simulink model "MdXXArray"  (R2024b)
settings: Solver=FixedStepDiscrete  StartTime=0.0  StopTime=10.0  FixedStep=0.01  RelTol=1e-3
(part 2 of 2)

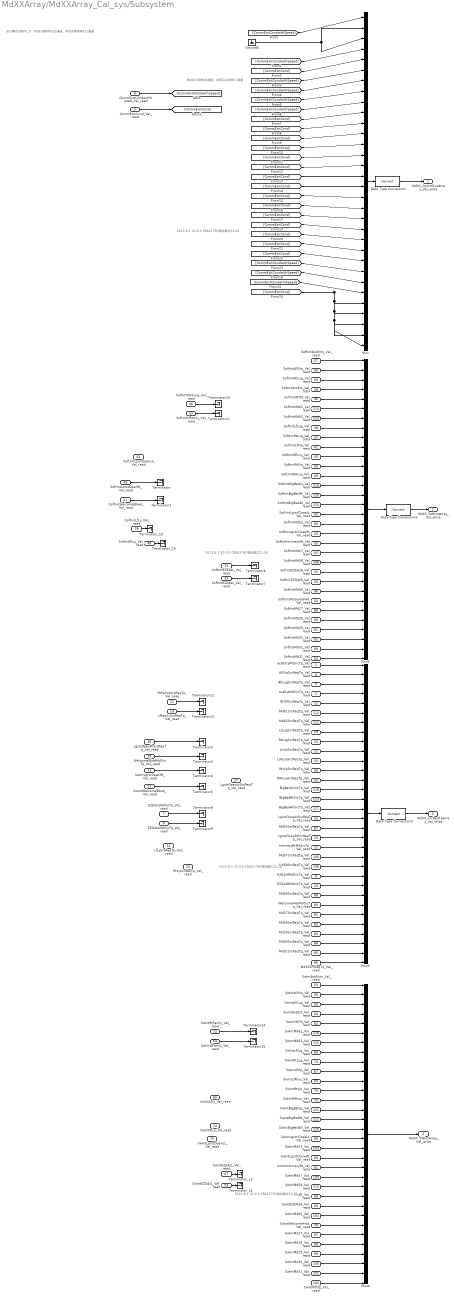
== system MdXXArray/MdXXArray_Cal_sys/Subsystem ==
  note: Md60占用Md6通道，Md61占用Md7通道
  note: 557模式流程V1.9：Md53借用Md18通道，Md56借用Md25通道
  note: 2023.8.1 V2.0.0 CR401790 增加模式21-26
  note: 2023.8.1 V2.0.0 CR401790 增加模式21-26
  note: 2023.8.1 V2.0.0 CR401790 增加模式21-26
  note: 2023.8.1 V2.0.0 CR421790 增加模式21-26
  acsEntyMdSrcTp_Val_read : Inport
  acsExtMdSrcTp_Val_read : Inport  Port=2
  AllLugSrcReqTp_Val_read : Inport  Port=3
  AllVipSrcReqTp_Val_read : Inport  Port=4
  CommExitCond_Val_read : Inport  Port=5
  CommExitCondwithSpeed_Val_read : Inport  Port=6
  EZE4sLMdSrcTp_Val_read : Inport  Port=7
  EZE4sRMdSrcTp_Val_read : Inport  Port=8
  EZQ4sLMdSrcTp_Val_read : Inport  Port=9
  EZQ4sRMdSrcTp_Val_read : Inport  Port=10
  IntimacyRtMdSrcTp_Val_read : Inport  Port=11
  INTMSrcReqTp_Val_read : Inport  Port=12
  LfFamlySrcReqTp_Val_read : Inport  Port=13
  LfLySrcReqTp_Val_read : Inport  Port=14
  LgrstCloseLtSrcReqTp_Val_read : Inport  Port=15
  LgrstCloseRtSrcReqTp_Val_read : Inport  Port=16
  LgrstOpenLtSrcReqTp_Val_read : Inport  Port=17
  LgrstOpenRtSrcReqTp_Val_read : Inport  Port=18
  LtLugSrcReqTp_Val_read : Inport  Port=19
  LtRcvySrcReqTp_Val_read : Inport  Port=20
  LtVipSrcReqTp_Val_read : Inport  Port=21
  RtFamlySrcReqTp_Val_read : Inport  Port=22
  RtLugSrcReqTp_Val_read : Inport  Port=23
  RtLySrcReqTp_Val_read : Inport  Port=24
  RtRcvySrcReqTp_Val_read : Inport  Port=25
  RtVipSrcReqTp_Val_read : Inport  Port=26
  SoftIntAcsEnty_Val_read : Inport  Port=27
  SoftIntAcsExt_Val_read : Inport  Port=28
  SoftIntAllLug_Val_read : Inport  Port=29
  SoftIntAllVip_Val_read : Inport  Port=30
  SoftIntEZE4sL_Val_read : Inport  Port=31
  SoftIntEZE4sR_Val_read : Inport  Port=32
  SoftIntEZQ4sL_Val_read : Inport  Port=33
  SoftIntEZQ4sR_Val_read : Inport  Port=34
  SoftIntIntimacyRt_Val_read : Inport  Port=35
  SoftIntINTM_Val_read : Inport  Port=36
  SoftIntLfFamly_Val_read : Inport  Port=37
  SoftIntLfLug_Val_read : Inport  Port=38
  SoftIntLfLy_Val_read : Inport  Port=39
  SoftIntLfRcvy_Val_read : Inport  Port=40
  SoftIntLfVip_Val_read : Inport  Port=41
  SoftIntLgrstCloseLt_Val_read : Inport  Port=42
  SoftIntLgrstCloseRt_Val_read : Inport  Port=43
  SoftIntLgrstOpenLt_Val_read : Inport  Port=44
  SoftIntLgrstOpenRt_Val_read : Inport  Port=45
  SoftIntRtFamly_Val_read : Inport  Port=46
  SoftIntRtLug_Val_read : Inport  Port=47
  SoftIntRtLy_Val_read : Inport  Port=48
  SoftIntRtRcvy_Val_read : Inport  Port=49
  SoftIntRtVip_Val_read : Inport  Port=50
  SoftIntWelcomeBkwd_Val_read : Inport  Port=51
  SoftIntWelcomeFwd_Val_read : Inport  Port=52
  SwIntAcsEnty_Val_read : Inport  Port=53
  SwIntAcsExt_Val_read : Inport  Port=54
  SwIntAllLug_Val_read : Inport  Port=55
  SwIntAllVip_Val_read : Inport  Port=56
  SwIntEZE4sL_Val_read : Inport  Port=57
  SwIntEZE4sR_Val_read : Inport  Port=58
  SwIntEZQ4sL_Val_read : Inport  Port=59
  SwIntEZQ4sR_Val_read : Inport  Port=60
  SwIntIntimacyRt_Val_read : Inport  Port=61
  SwIntINTM_Val_read : Inport  Port=62
  SwIntLfFamly_Val_read : Inport  Port=63
  SwIntLfLug_Val_read : Inport  Port=64
  SwIntLfLy_Val_read : Inport  Port=65
  SwIntLfRcvy_Val_read : Inport  Port=66
  SwIntLfVip_Val_read : Inport  Port=67
  SwIntLgrstCloseLt_Val_read : Inport  Port=68
  SwIntLgrstCloseRt_Val_read : Inport  Port=69
  SwIntLgrstOpenLt_Val_read : Inport  Port=70
  SwIntLgrstOpenRt_Val_read : Inport  Port=71
  SwIntRtFamly_Val_read : Inport  Port=72
  SwIntRtLug_Val_read : Inport  Port=73
  SwIntRtLy_Val_read : Inport  Port=74
  SwIntRtRcvy_Val_read : Inport  Port=75
  SwIntRtVip_Val_read : Inport  Port=76
  SwIntWelcomeBkwd_Val_read : Inport  Port=77
  SwIntWelcomeFwd_Val_read : Inport  Port=78
  WelcomeBkwdMdSrcTp_Val_read : Inport  Port=79
  WelcomeFwdMdSrcTp_Val_read : Inport  Port=80
  Md27SrcReqTp_Val_read : Inport  Port=81
  Md28SrcReqTp_Val_read : Inport  Port=82
  Md29SrcReqTp_Val_read : Inport  Port=83
  Md30SrcReqTp_Val_read : Inport  Port=84
  Md31SrcReqTp_Val_read : Inport  Port=85
  Md32SrcReqTp_Val_read : Inport  Port=86
  Md53SrcReqTp_Val_read : Inport  Port=87
  Md56SrcReqTp_Val_read : Inport  Port=88
  SoftIntMd27_Val_read : Inport  Port=89
  SoftIntMd28_Val_read : Inport  Port=90
  SoftIntMd29_Val_read : Inport  Port=91
  SoftIntMd30_Val_read : Inport  Port=92
  SoftIntMd31_Val_read : Inport  Port=93
  SoftIntMd32_Val_read : Inport  Port=94
  SoftIntMd53_Val_read : Inport  Port=95
  SoftIntMd56_Val_read : Inport  Port=96
  SwIntMd27_Val_read : Inport  Port=97
  SwIntMd28_Val_read : Inport  Port=98
  SwIntMd29_Val_read : Inport  Port=99
  SwIntMd30_Val_read : Inport  Port=100
  SwIntMd31_Val_read : Inport  Port=101
  SwIntMd32_Val_read : Inport  Port=102
  SwIntMd53_Val_read : Inport  Port=103
  SwIntMd56_Val_read : Inport  Port=104
  Md57SrcReqTp_Val_read : Inport  Port=105
  Md58SrcReqTp_Val_read : Inport  Port=106
  SoftIntMd57_Val_read : Inport  Port=107
  SoftIntMd58_Val_read : Inport  Port=108
  SwIntMd57_Val_read : Inport  Port=109
  SwIntMd58_Val_read : Inport  Port=110
  Md62SrcReqTp_Val_read : Inport  Port=111
  Md61SrcReqTp_Val_read : Inport  Port=112
  SoftIntMd62_Val_read : Inport  Port=113
  SoftIntMd61_Val_read : Inport  Port=114
  SwIntMd62_Val_read : Inport  Port=115
  SwIntMd61_Val_read : Inport  Port=116
  BigBedAllSrcTp_Val_read : Inport  Port=117
  BigBedLtSrcTp_Val_read : Inport  Port=118
  SoftIntBigBedLt_Val_read : Inport  Port=119
  SwIntBigBedAll_Val_read : Inport  Port=120
  SwIntBigBedLt_Val_read : Inport  Port=121
  SwIntBigBedRt_Val_read : Inport  Port=122
  BigBedRtSrcTp_Val_read : Inport  Port=123
  SoftIntBigBedAll_Val_read : Inport  Port=124
  SoftIntBigBedRt_Val_read : Inport  Port=125
  Data Type Conversion : DataTypeConversion  SaturateOnIntegerOverflow=off  RndMeth=Floor
  Data Type Conversion2 : DataTypeConversion  SaturateOnIntegerOverflow=off  RndMeth=Floor
  Data Type Conversion3 : DataTypeConversion  SaturateOnIntegerOverflow=off  RndMeth=Floor
  Ground5 : Ground
  Mux{,2..4} (4 alike) : Mux  Inputs=32
  Terminator{,1..15} (16 alike) : Terminator
  Terminator_{13..14,19..20} (4 alike) : Terminator
  MdXX_CommExitArray_Val_write : Outport  VectorParamsAs1DForOutWhenUnconnected=off
      settings: EnsureOutportIsVirtual=on
  MdXX_SoftIntArray_Val_write : Outport  Port=2  VectorParamsAs1DForOutWhenUnconnected=off
      settings: EnsureOutportIsVirtual=on
  MdXX_SrcReqTpArray_Val_write : Outport  Port=3  VectorParamsAs1DForOutWhenUnconnected=off
      settings: EnsureOutportIsVirtual=on
  MdXX_SWIntArray_Val_write : Outport  Port=4  VectorParamsAs1DForOutWhenUnconnected=off
      settings: EnsureOutportIsVirtual=on
  wires:
  CommExitCondwithSpeed_Val_read/1 -> [CommExitCondwithSpeed]
  Mux4/1 -> MdXX_SWIntArray_Val_write/1
  Mux2/1 -> Data Type Conversion2/1
  Mux3/1 -> Data Type Conversion3/1
  SoftIntAcsEnty_Val_read/1 -> Mux2/1
  SoftIntAllVip_Val_read/1 -> Mux2/2
  SoftIntAllLug_Val_read/1 -> Mux2/3
  SoftIntAcsExt_Val_read/1 -> Mux2/4
  SoftIntINTM_Val_read/1 -> Mux2/5
  SoftIntLfLug_Val_read/1 -> Mux2/8
  SoftIntRtLug_Val_read/1 -> Mux2/9
  SoftIntLfVip_Val_read/1 -> Mux2/10
  SoftIntLfRcvy_Val_read/1 -> Mux2/11
  SoftIntRtVip_Val_read/1 -> Mux2/12
  SoftIntRtRcvy_Val_read/1 -> Mux2/13
  SoftIntLgrstCloseLt_Val_read/1 -> Mux2/17
  SoftIntLgrstCloseRt_Val_read/1 -> Mux2/19
  SoftIntIntimacyRt_Val_read/1 -> Mux2/20
  SoftIntEZE4sR_Val_read/1 -> Mux2/23
  SoftIntEZQ4sR_Val_read/1 -> Mux2/24
  SoftIntWelcomeFwd_Val_read/1 -> Mux2/26
  acsEntyMdSrcTp_Val_read/1 -> Mux3/1
  AllVipSrcReqTp_Val_read/1 -> Mux3/2
  AllLugSrcReqTp_Val_read/1 -> Mux3/3
  acsExtMdSrcTp_Val_read/1 -> Mux3/4
  INTMSrcReqTp_Val_read/1 -> Mux3/5
  LtLugSrcReqTp_Val_read/1 -> Mux3/8
  RtLugSrcReqTp_Val_read/1 -> Mux3/9
  LtVipSrcReqTp_Val_read/1 -> Mux3/10
  LtRcvySrcReqTp_Val_read/1 -> Mux3/11
  RtVipSrcReqTp_Val_read/1 -> Mux3/12
  RtRcvySrcReqTp_Val_read/1 -> Mux3/13
  LgrstCloseLtSrcReqTp_Val_read/1 -> Mux3/17
  LgrstCloseRtSrcReqTp_Val_read/1 -> Mux3/19
  IntimacyRtMdSrcTp_Val_read/1 -> Mux3/20
  EZE4sRMdSrcTp_Val_read/1 -> Mux3/23
  EZQ4sRMdSrcTp_Val_read/1 -> Mux3/24
  WelcomeFwdMdSrcTp_Val_read/1 -> Mux3/26
  SwIntAcsEnty_Val_read/1 -> Mux4/1
  SwIntAllVip_Val_read/1 -> Mux4/2
  SwIntAllLug_Val_read/1 -> Mux4/3
  SwIntAcsExt_Val_read/1 -> Mux4/4
  SwIntINTM_Val_read/1 -> Mux4/5
  SwIntLfLug_Val_read/1 -> Mux4/8
  SwIntRtLug_Val_read/1 -> Mux4/9
  SwIntLfVip_Val_read/1 -> Mux4/10
  SwIntLfRcvy_Val_read/1 -> Mux4/11
  SwIntRtVip_Val_read/1 -> Mux4/12
  SwIntRtRcvy_Val_read/1 -> Mux4/13
  SwIntLgrstCloseLt_Val_read/1 -> Mux4/17
  SwIntLgrstCloseRt_Val_read/1 -> Mux4/19
  SwIntIntimacyRt_Val_read/1 -> Mux4/20
  SwIntEZE4sR_Val_read/1 -> Mux4/23
  SwIntEZQ4sR_Val_read/1 -> Mux4/24
  SwIntWelcomeFwd_Val_read/1 -> Mux4/26
  CommExitCond_Val_read/1 -> [CommExitCond]
  [CommExitCondwithSpeed] -> Mux/1
  [CommExitCondwithSpeed] -> Mux/4
  Ground5/1 -> Mux/3, Mux/2
  [CommExitCond] -> Mux/5
  [CommExitCondwithSpeed] -> Mux/8
  [CommExitCondwithSpeed] -> Mux/9
  [CommExitCond] -> Mux/10
  [CommExitCond] -> Mux/11
  [CommExitCond] -> Mux/12
  [CommExitCond] -> Mux/13
  [CommExitCond] -> Mux/14
  [CommExitCond] -> Mux/15
  [CommExitCond] -> Mux/16
  [CommExitCond] -> Mux/17
  [CommExitCond] -> Mux/18
  [CommExitCond] -> Mux/19
  [CommExitCond] -> Mux/28, Mux/29, Mux/30, Mux/32, Mux/31
  [CommExitCond] -> Mux/20
  [CommExitCondwithSpeed] -> Mux/26
  [CommExitCond] -> Mux/21
  [CommExitCond] -> Mux/22
  [CommExitCond] -> Mux/23
  [CommExitCond] -> Mux/24
  [CommExitCondwithSpeed] -> Mux/25
  Mux/1 -> Data Type Conversion/1
  Data Type Conversion/1 -> MdXX_CommExitArray_Val_write/1
  Data Type Conversion2/1 -> MdXX_SoftIntArray_Val_write/1
  Data Type Conversion3/1 -> MdXX_SrcReqTpArray_Val_write/1
  SoftIntMd27_Val_read/1 -> Mux2/27
  SoftIntMd28_Val_read/1 -> Mux2/28
  SoftIntMd29_Val_read/1 -> Mux2/29
  SoftIntMd30_Val_read/1 -> Mux2/30
  SoftIntMd31_Val_read/1 -> Mux2/31
  SoftIntMd32_Val_read/1 -> Mux2/32
  SoftIntMd53_Val_read/1 -> Mux2/18
  SoftIntMd56_Val_read/1 -> Mux2/25
  SoftIntLgrstOpenRt_Val_read/1 -> Terminator/1
  SoftIntWelcomeBkwd_Val_read/1 -> Terminator1/1
  Md53SrcReqTp_Val_read/1 -> Mux3/18
  Md56SrcReqTp_Val_read/1 -> Mux3/25
  Md27SrcReqTp_Val_read/1 -> Mux3/27
  Md28SrcReqTp_Val_read/1 -> Mux3/28
  Md29SrcReqTp_Val_read/1 -> Mux3/29
  Md30SrcReqTp_Val_read/1 -> Mux3/30
  Md31SrcReqTp_Val_read/1 -> Mux3/31
  Md32SrcReqTp_Val_read/1 -> Mux3/32
  SwIntMd27_Val_read/1 -> Mux4/27
  SwIntMd28_Val_read/1 -> Mux4/28
  SwIntMd29_Val_read/1 -> Mux4/29
  SwIntMd30_Val_read/1 -> Mux4/30
  SwIntMd31_Val_read/1 -> Mux4/31
  SwIntMd32_Val_read/1 -> Mux4/32
  SwIntMd56_Val_read/1 -> Mux4/25
  SwIntMd53_Val_read/1 -> Mux4/18
  LgrstOpenRtSrcReqTp_Val_read/1 -> Terminator2/1
  WelcomeBkwdMdSrcTp_Val_read/1 -> Terminator3/1
  SwIntLgrstOpenRt_Val_read/1 -> Terminator4/1
  SwIntWelcomeBkwd_Val_read/1 -> Terminator5/1
  SoftIntMd57_Val_read/1 -> Mux2/21
  SoftIntMd58_Val_read/1 -> Mux2/22
  SwIntMd57_Val_read/1 -> Mux4/21
  SwIntMd58_Val_read/1 -> Mux4/22
  SoftIntEZE4sL_Val_read/1 -> Terminator6/1
  SoftIntEZQ4sL_Val_read/1 -> Terminator7/1
  EZE4sLMdSrcTp_Val_read/1 -> Terminator8/1
  EZQ4sLMdSrcTp_Val_read/1 -> Terminator9/1
  Md57SrcReqTp_Val_read/1 -> Mux3/21
  Md58SrcReqTp_Val_read/1 -> Mux3/22
  [CommExitCondwithSpeed] -> Mux/6
  [CommExitCondwithSpeed] -> Mux/7
  SoftIntRtFamly_Val_read/1 -> Terminator10/1
  SoftIntLfFamly_Val_read/1 -> Terminator11/1
  SwIntEZE4sL_Val_read/1 -> Terminator_13/1
  SwIntEZQ4sL_Val_read/1 -> Terminator_14/1
  RtFamlySrcReqTp_Val_read/1 -> Terminator12/1
  LfFamlySrcReqTp_Val_read/1 -> Terminator13/1
  SwIntRtFamly_Val_read/1 -> Terminator14/1
  SwIntLfFamly_Val_read/1 -> Terminator15/1
  SoftIntMd61_Val_read/1 -> Mux2/6
  SoftIntMd62_Val_read/1 -> Mux2/7
  Md61SrcReqTp_Val_read/1 -> Mux3/6
  Md62SrcReqTp_Val_read/1 -> Mux3/7
  SwIntMd61_Val_read/1 -> Mux4/6
  SwIntMd62_Val_read/1 -> Mux4/7
  SoftIntBigBedLt_Val_read/1 -> Mux2/14
  SoftIntLfLy_Val_read/1 -> Terminator_19/1
  SoftIntRtLy_Val_read/1 -> Terminator_20/1
  BigBedLtSrcTp_Val_read/1 -> Mux3/14
  SwIntBigBedAll_Val_read/1 -> Mux4/16
  SwIntBigBedRt_Val_read/1 -> Mux4/15
  SoftIntBigBedRt_Val_read/1 -> Mux2/15
  SoftIntBigBedAll_Val_read/1 -> Mux2/16
  BigBedRtSrcTp_Val_read/1 -> Mux3/15
  BigBedAllSrcTp_Val_read/1 -> Mux3/16
  SwIntBigBedLt_Val_read/1 -> Mux4/14
  [CommExitCondwithSpeed] -> Mux/27
